simulink model "EKF"  (R2016a)
settings: Solver=VariableStepAuto  StartTime=0.0  StopTime=10.0  RelTol=1e-3
values from neighbouring files (symbols this model uses):
  uk = Fin(Noutput+1:Noutput+Ninput)    [ExKalmanFilter.m]
  Ymeas = Fin(1:Noutput)    [ExKalmanFilter.m]
settings Model: Creator=hp  LastModifiedBy=hp

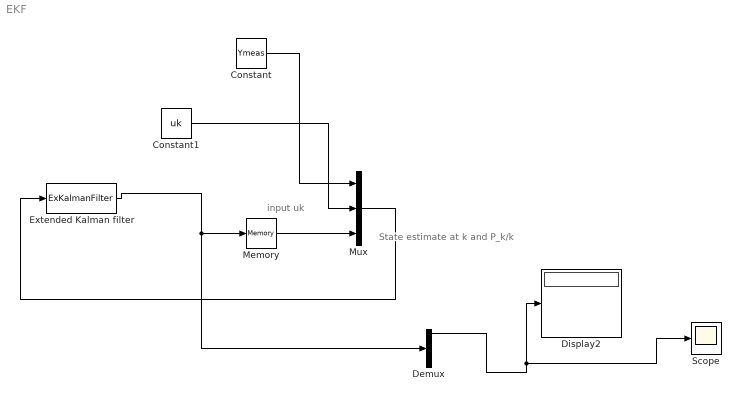
== system EKF ==
  note: input uk
  note: State estimate at k and P_k/k
  Constant : Constant  Value=Ymeas
  Constant1 : Constant  Value=uk
  Demux : Demux
  Display2 : Display
      settings: Decimation=3
  Extended Kalman filter : MATLABFcn  MATLABFcn=ExKalmanFilter  OutputDimensions=12
  Memory : Memory  X0=Fin(5:end)
  Mux : Mux  Inputs=3
  Scope : Scope
  wires:
  Mux/1 -> Extended Kalman filter/1
  Extended Kalman filter/1 -> Demux/1, Memory/1
  Memory/1 -> Mux/3
  Demux/1 -> Scope/1, Display2/1
  Constant1/1 -> Mux/2
  Constant/1 -> Mux/1
